simulink model "zad3"  (R2017b)
settings: Solver=VariableStepAuto  StartTime=0.0  StopTime=0  RelTol=1e-3
libraries: CPOiS_SourcesSinks x10, CPOiS_LinearTransforms x8, CPOiS_DataManipulation_DataTypeConversion x6, CPOiS_Filters x4, CPOiS_General x1
settings Model: Creator=kstefanc  LastModifiedBy=kstefanc

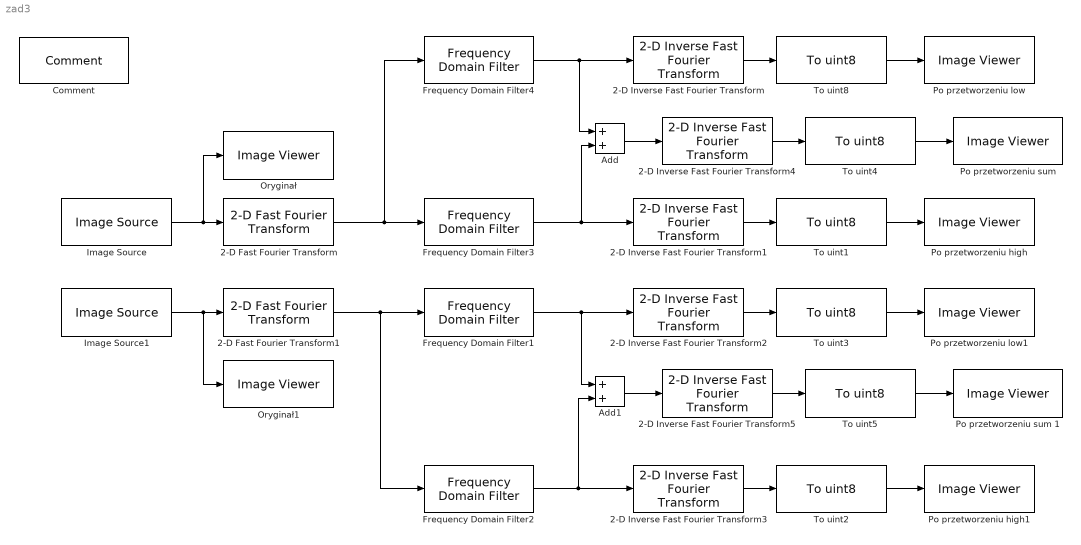
== system zad3 ==
  2-D Fast Fourier Transform : CPOiS_LinearTransforms/2-D Fast Fourier Transform
      settings: SourceProductName=CPOiS - Digital image and signal processing
  2-D Fast Fourier Transform1 : CPOiS_LinearTransforms/2-D Fast Fourier Transform
      settings: SourceProductName=CPOiS - Digital image and signal processing
  2-D Inverse Fast Fourier Transform{,1..5} (6 alike) : CPOiS_LinearTransforms/2-D Inverse Fast  Fourier Transform
      settings: SourceProductName=CPOiS - Digital image and signal processing
  Add : Sum
  Add1 : Sum
  Comment : CPOiS_General/Comment
      settings: SourceProductName=CPOiS - Digital image and signal processing
  Frequency Domain Filter1 : CPOiS_Filters/Frequency Domain Filter  filtertype=Low-pass Filter  radius=10
      settings: SourceProductName=CPOiS - Digital image and signal processing
  Frequency Domain Filter2 : CPOiS_Filters/Frequency Domain Filter  filtertype=High-pass Filter  radius=10
      settings: SourceProductName=CPOiS - Digital image and signal processing
  Frequency Domain Filter3 : CPOiS_Filters/Frequency Domain Filter  filtertype=High-pass Filter  radius=10
      settings: SourceProductName=CPOiS - Digital image and signal processing
  Frequency Domain Filter4 : CPOiS_Filters/Frequency Domain Filter  filtertype=Low-pass Filter  radius=10
      settings: SourceProductName=CPOiS - Digital image and signal processing
  Image Source : CPOiS_SourcesSinks/Image Source  FileSelection=gull.png
      settings: SourceProductName=CPOiS - Digital image and signal processing
  Image Source1 : CPOiS_SourcesSinks/Image Source  FileSelection=ball.png
      settings: SourceProductName=CPOiS - Digital image and signal processing
  Oryginał : CPOiS_SourcesSinks/Image Viewer
      settings: SourceProductName=CPOiS - Digital image and signal processing
  Oryginał1 : CPOiS_SourcesSinks/Image Viewer
      settings: SourceProductName=CPOiS - Digital image and signal processing
  Po przetworzeniu high : CPOiS_SourcesSinks/Image Viewer
      settings: SourceProductName=CPOiS - Digital image and signal processing
  "Po przetworzeniu high1 " : CPOiS_SourcesSinks/Image Viewer
      settings: SourceProductName=CPOiS - Digital image and signal processing
  Po przetworzeniu low : CPOiS_SourcesSinks/Image Viewer
      settings: SourceProductName=CPOiS - Digital image and signal processing
  Po przetworzeniu low1 : CPOiS_SourcesSinks/Image Viewer
      settings: SourceProductName=CPOiS - Digital image and signal processing
  "Po przetworzeniu sum " : CPOiS_SourcesSinks/Image Viewer
      settings: SourceProductName=CPOiS - Digital image and signal processing
  Po przetworzeniu sum 1 : CPOiS_SourcesSinks/Image Viewer
      settings: SourceProductName=CPOiS - Digital image and signal processing
  To uint{1..5,8} (6 alike) : CPOiS_DataManipulation_DataTypeConversion/To uint8
      settings: SourceProductName=CPOiS - Digital image and signal processing
  wires:
  Image Source/1 -> 2-D Fast Fourier Transform/1, Oryginał/1
  2-D Inverse Fast Fourier Transform/1 -> To uint8/1
  To uint8/1 -> Po przetworzeniu low/1
  2-D Inverse Fast Fourier Transform1/1 -> To uint1/1
  Image Source1/1 -> 2-D Fast Fourier Transform1/1, Oryginał1/1
  To uint1/1 -> Po przetworzeniu high/1
  To uint2/1 -> "Po przetworzeniu high1 "/1
  2-D Inverse Fast Fourier Transform2/1 -> To uint3/1
  To uint3/1 -> Po przetworzeniu low1/1
  2-D Inverse Fast Fourier Transform3/1 -> To uint2/1
  2-D Fast Fourier Transform/1 -> Frequency Domain Filter4/1, Frequency Domain Filter3/1
  2-D Fast Fourier Transform1/1 -> Frequency Domain Filter2/1, Frequency Domain Filter1/1
  Frequency Domain Filter4/1 -> Add/1, 2-D Inverse Fast Fourier Transform/1
  Frequency Domain Filter3/1 -> Add/2, 2-D Inverse Fast Fourier Transform1/1
  Frequency Domain Filter1/1 -> Add1/1, 2-D Inverse Fast Fourier Transform2/1
  Frequency Domain Filter2/1 -> Add1/2, 2-D Inverse Fast Fourier Transform3/1
  Add/1 -> 2-D Inverse Fast Fourier Transform4/1
  Add1/1 -> 2-D Inverse Fast Fourier Transform5/1
  To uint5/1 -> Po przetworzeniu sum 1/1
  2-D Inverse Fast Fourier Transform5/1 -> To uint5/1
  2-D Inverse Fast Fourier Transform4/1 -> To uint4/1
  To uint4/1 -> "Po przetworzeniu sum "/1
